simulink model "vehicleModel"  (R2022a)
settings: Solver=ode4  StartTime=0.0  StopTime=100  FixedStep=0.01  RelTol=1e-3
model workspace (MAT data in the model file):
  K = 1
  N = [1 1]
  X = 1
(part 1 of 2)
settings Model: Creator=82106  LastModifiedBy=user
settings ModelReferenceCC: EnableRefExpFcnMdlSchedulingChecks=off
settings RTWCC: Description=Generic Real-Time Target

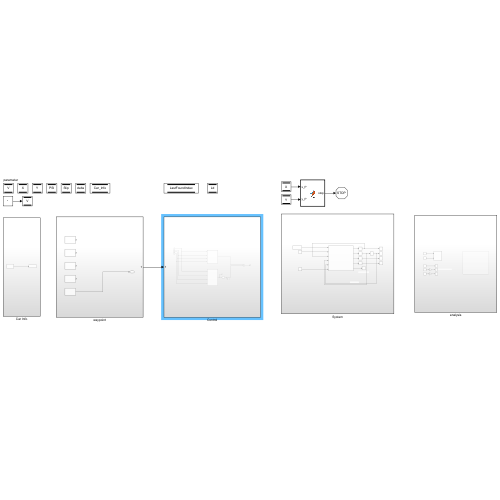
[thumbnail: Simulink's stored preview of the top-level diagram]
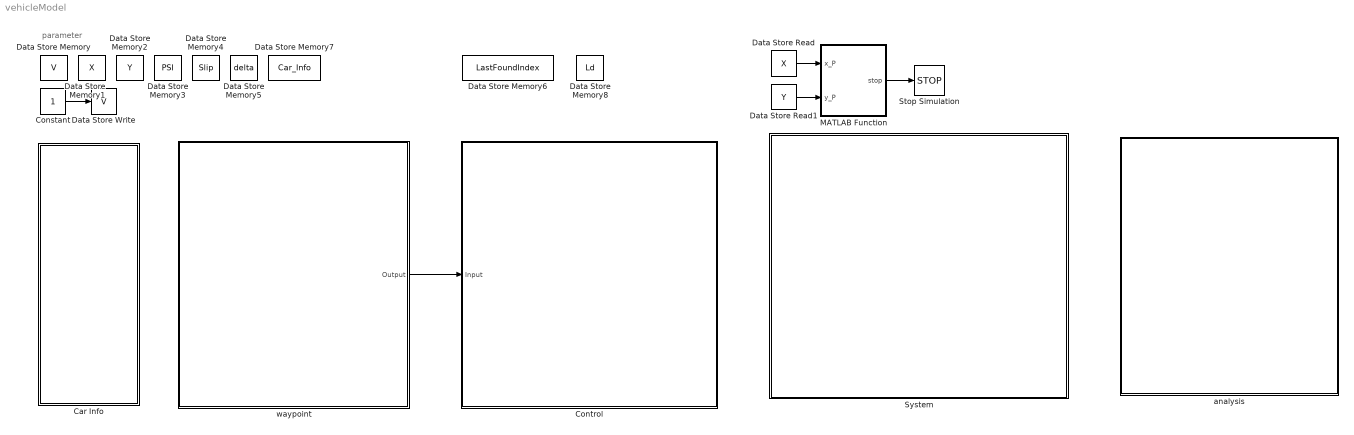
== system vehicleModel ==
  note: parameter
  Car Info : Subsystem
  Constant : Constant
  Control : Subsystem
  Data Store Memory : DataStoreMemory  DataStoreName=V  WriteAfterWriteMsg=warning  ShowAdditionalParam=off
  Data Store Memory1 : DataStoreMemory  DataStoreName=X  WriteAfterWriteMsg=warning  ShowAdditionalParam=off
  Data Store Memory2 : DataStoreMemory  DataStoreName=Y  WriteAfterWriteMsg=warning  ShowAdditionalParam=off
  Data Store Memory3 : DataStoreMemory  DataStoreName=PSI  WriteAfterWriteMsg=warning  ShowAdditionalParam=off
  Data Store Memory4 : DataStoreMemory  DataStoreName=Slip  WriteAfterWriteMsg=warning  ShowAdditionalParam=off
  Data Store Memory5 : DataStoreMemory  DataStoreName=delta  WriteAfterWriteMsg=warning  ShowAdditionalParam=off
  Data Store Memory6 : DataStoreMemory  DataStoreName=LastFoundIndex  WriteAfterWriteMsg=warning  InitialValue=1  ShowAdditionalParam=off
  Data Store Memory7 : DataStoreMemory  DataStoreName=Car_Info  WriteAfterWriteMsg=warning  ShowAdditionalParam=off  Dimensions=6
  Data Store Memory8 : DataStoreMemory  DataStoreName=Ld  WriteAfterWriteMsg=warning  InitialValue=3  ShowAdditionalParam=off
  Data Store Read : DataStoreRead  DataStoreName=X  IndexOptions=Index vector (dialog)  Indices=1  OutputSizes=1
  Data Store Read1 : DataStoreRead  DataStoreName=Y  IndexOptions=Index vector (dialog)  Indices=1  OutputSizes=1
  Data Store Write : DataStoreWrite  DataStoreName=V  IndexOptions=Index vector (dialog)  Indices=1  OutputSizes=1
  MATLAB Function : MATLAB Function  TreatAsAtomicUnit=on
  Stop Simulation : Stop
  System : Subsystem
  analysis : Subsystem
  waypoint : Subsystem
  wires:
  Constant/1 -> Data Store Write/1
  waypoint/1(Output) -> Control/1(Input)
  Data Store Read/1 -> MATLAB Function/1(x_P)
  MATLAB Function/1(stop) -> Stop Simulation/1
  Data Store Read1/1 -> MATLAB Function/2(y_P)

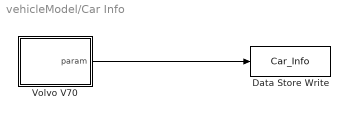
== system vehicleModel/Car Info ==
  Data Store Write : DataStoreWrite  DataStoreName=Car_Info  IndexOptions=Index vector (dialog)  Indices=1  OutputSizes=1
  Volvo V70 : MATLAB Function  TreatAsAtomicUnit=on
  wires:
  Volvo V70/1(param) -> Data Store Write/1

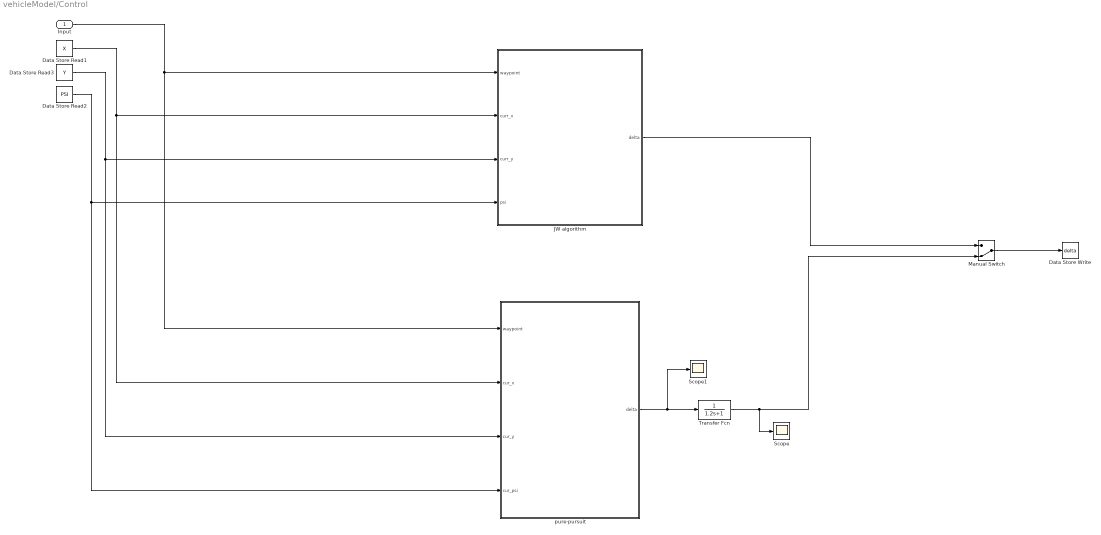
== system vehicleModel/Control ==
  Input : Inport
  Data Store Read1 : DataStoreRead  DataStoreName=X  IndexOptions=Index vector (dialog)  Indices=1  OutputSizes=1
  Data Store Read2 : DataStoreRead  DataStoreName=PSI  IndexOptions=Index vector (dialog)  Indices=1  OutputSizes=1
  Data Store Read3 : DataStoreRead  DataStoreName=Y  IndexOptions=Index vector (dialog)  Indices=1  OutputSizes=1
  Data Store Write : DataStoreWrite  DataStoreName=delta  IndexOptions=Index vector (dialog)  Indices=1  OutputSizes=1
  JW algorithm : Subsystem
  Manual Switch : ManualSwitch  CurrentSetting=0
  Scope : Scope
  Scope1 : Scope
  Transfer Fcn : TransferFcn  Denominator=[1.2 1]
  pure-pursuit : Subsystem
  wires:
  Input/1 -> pure-pursuit/1(waypoint), JW algorithm/1(waypoint)
  Data Store Read2/1 -> pure-pursuit/4(cur_psi), JW algorithm/4(psi)
  Data Store Read3/1 -> pure-pursuit/3(cur_y), JW algorithm/3(curr_y)
  Data Store Read1/1 -> pure-pursuit/2(cur_x), JW algorithm/2(curr_x)
  JW algorithm/1(delta) -> Manual Switch/1
  pure-pursuit/1(delta) -> Scope1/1, Transfer Fcn/1
  Manual Switch/1 -> Data Store Write/1
  Transfer Fcn/1 -> Scope/1, Manual Switch/2

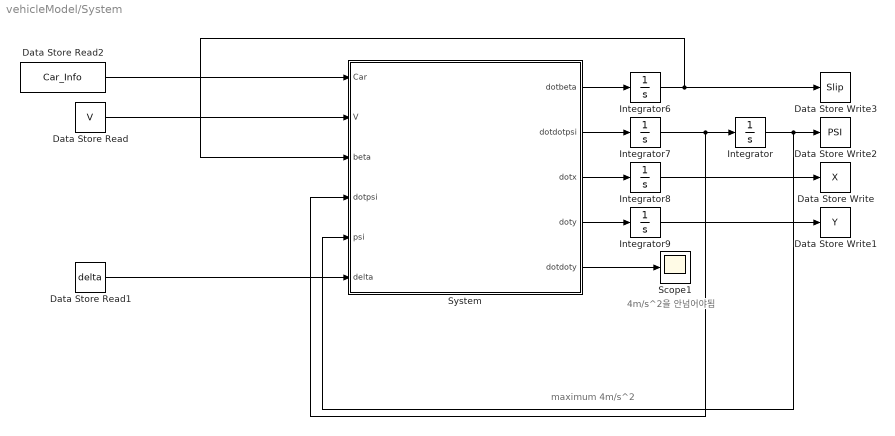
== system vehicleModel/System ==
  note: 4m/s^2을 안넘어야됨
  note: maximum 4m/s^2
  Data Store Read : DataStoreRead  DataStoreName=V  IndexOptions=Index vector (dialog)  Indices=1  OutputSizes=1
  Data Store Read1 : DataStoreRead  DataStoreName=delta  IndexOptions=Index vector (dialog)  Indices=1  OutputSizes=1
  Data Store Read2 : DataStoreRead  DataStoreName=Car_Info  IndexOptions=Index vector (dialog)  Indices=1  OutputSizes=1
  Data Store Write : DataStoreWrite  DataStoreName=X  IndexOptions=Index vector (dialog)  Indices=1  OutputSizes=1
  Data Store Write1 : DataStoreWrite  DataStoreName=Y  IndexOptions=Index vector (dialog)  Indices=1  OutputSizes=1
  Data Store Write2 : DataStoreWrite  DataStoreName=PSI  IndexOptions=Index vector (dialog)  Indices=1  OutputSizes=1
  Data Store Write3 : DataStoreWrite  DataStoreName=Slip  IndexOptions=Index vector (dialog)  Indices=1  OutputSizes=1
  Integrator : Integrator
  Integrator6 : Integrator
  Integrator7 : Integrator
  Integrator8 : Integrator  InitialCondition=1
  Integrator9 : Integrator  InitialCondition=1
  Scope1 : Scope
  System : MATLAB Function  TreatAsAtomicUnit=on
  wires:
  System/5(dotdoty) -> Scope1/1
  System/2(dotdotpsi) -> Integrator7/1
  Integrator9/1 -> Data Store Write1/1
  Integrator6/1 -> System/3(beta), Data Store Write3/1
  Data Store Read/1 -> System/2(V)
  Integrator/1 -> Data Store Write2/1, System/5(psi)
  System/4(doty) -> Integrator9/1
  System/3(dotx) -> Integrator8/1
  Integrator7/1 -> System/4(dotpsi), Integrator/1
  System/1(dotbeta) -> Integrator6/1
  Data Store Read2/1 -> System/1(Car)
  Integrator8/1 -> Data Store Write/1
  Data Store Read1/1 -> System/6(delta)

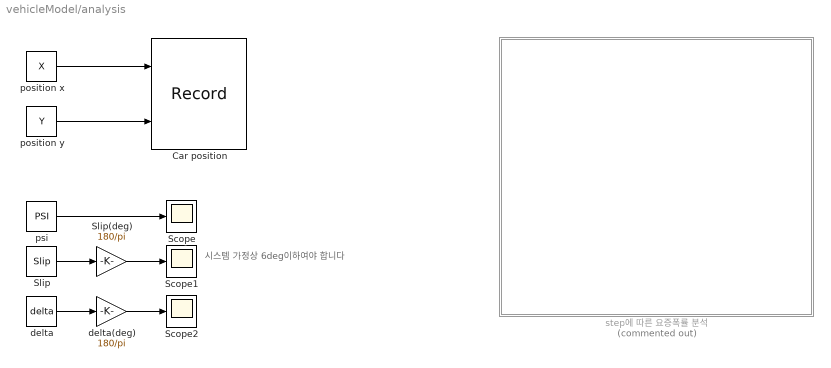
== system vehicleModel/analysis ==
  note: 시스템 가정상 6deg이하여야 합니다
  Car position : Record  FileSettingsInternal="{\"entries\":[{\"content\":{\"excelSettings\":{\"content\":{},\"type\":\"Streamout.ExcelSettings\"}},\"type\":\"Streamout.FileSettingStorage\",\"uuid\":\"dac2e031-e7b2-4fcf-a58f-8ca8c39981c0\"}],\"packageUris\":[\"http://schema.mathworks.com/mf0/streamout_blocks/R2020a\"],\"version\":\"1.0\"}"  Layout=[1 1]  SignalsInternal="{\"entries\":[{\"content\":{\"signals\":[{\"content\":{\"blockPath\":[\"vehicleModel/analysis/Car position\"],\"channel\":[],\"dimensions\":[1],\"domain\":\"vehicleModel/analysis/Car position\",\"lineColor\":\"#a2142f\",\"plots\":[],\"port\":1,\"sid\":[\"\"],\"signalID\":1105,\"signalName\":\"position x\"},\"type\":\"RecordBlkView.Signal\",\"uuid\":\"3ba0c8e4-d376-4e94-8844-daf1410684dd\"},{\"content\":{\"blockPath\":[\"vehicleModel/analysis/Car position\"],\"channel\":[],\"dimensions\":[1],\"domain\":\"vehicleModel/analysis/Car position\",\"lineColor\":\"#139fff\",\"plots\":[1],\"port\":2,\"sid\":[\"\"],\"signalID\":1109,\"signalName\":\"position y\"},\"type\":\"RecordBlkView.Signal\",\"uuid\":\"fbcaf7b4-362f-417e-84a3-3c3b3bc75f13\"}]},\"type\":\"RecordBlkView.InputSignals\",\"uuid\":\"d27d3567-7b96-48c0-b7eb-1a5b4245cb3a\"}],\"packageUris\":[\"http://schema.mathworks.com/mf0/streamout_blocks/R2020a\"],\"version\":\"1.0\"}"  VisualizationBindings="{\"xyplotplugin\":{\"info\":[{\"series\":[{\"bindingParametersList\":[{\"parameter\":\"Y-Axis\",\"signalID\":1109,\"signalName\":\"position y\"}],\"seriesID\":39458}],\"subplotID\":1}]}}"  CompatibilityTag=XY  st=-1
  Scope : Scope
  Scope1 : Scope
  Scope2 : Scope
  Slip : DataStoreRead  DataStoreName=Slip  IndexOptions=Index vector (dialog)  Indices=1  OutputSizes=1
  Slip(deg) : Gain  Gain=180/pi
  delta : DataStoreRead  DataStoreName=delta  IndexOptions=Index vector (dialog)  Indices=1  OutputSizes=1
  delta(deg) : Gain  Gain=180/pi
  position x : DataStoreRead  DataStoreName=X  IndexOptions=Index vector (dialog)  Indices=1  OutputSizes=1
  position y : DataStoreRead  DataStoreName=Y  IndexOptions=Index vector (dialog)  Indices=1  OutputSizes=1
  psi : DataStoreRead  DataStoreName=PSI  IndexOptions=Index vector (dialog)  Indices=1  OutputSizes=1
  step에 따른 요증폭률 분석 : Subsystem  Commented=on
  wires:
  position x/1 -> Car position/1
  position y/1 -> Car position/2
  psi/1 -> Scope/1
  Slip/1 -> Slip(deg)/1
  delta/1 -> delta(deg)/1
  Slip(deg)/1 -> Scope1/1
  delta(deg)/1 -> Scope2/1

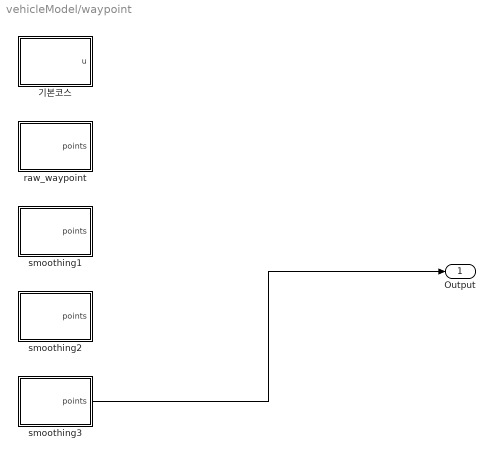
== system vehicleModel/waypoint ==
  raw_waypoint : MATLAB Function  TreatAsAtomicUnit=on
  smoothing1 : MATLAB Function  TreatAsAtomicUnit=on
  smoothing2 : MATLAB Function  TreatAsAtomicUnit=on
  smoothing3 : MATLAB Function  TreatAsAtomicUnit=on
  기본코스 : MATLAB Function  TreatAsAtomicUnit=on
  Output : Outport
  wires:
  smoothing3/1(points) -> Output/1

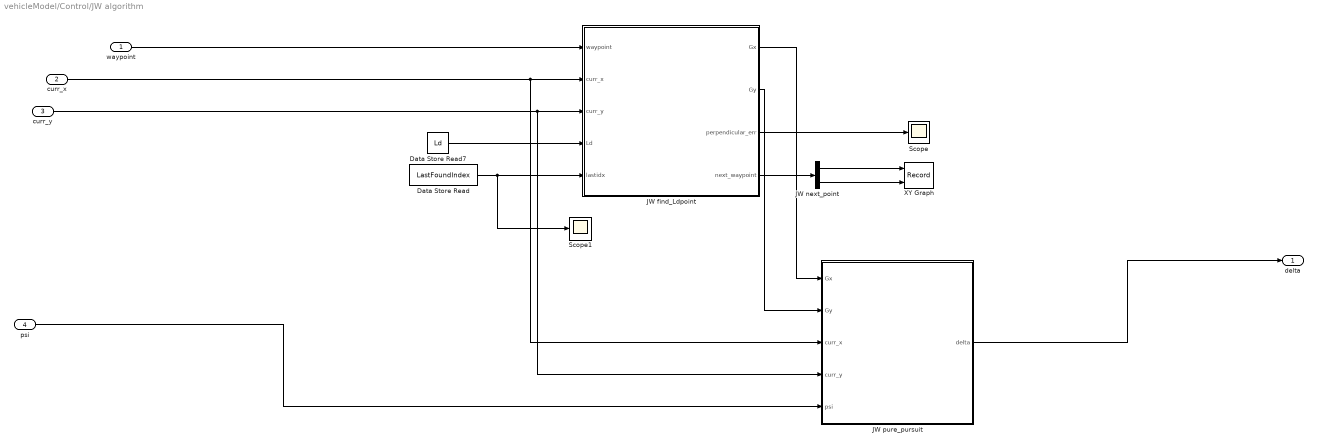
== system vehicleModel/Control/JW algorithm ==
  waypoint : Inport
  curr_x : Inport  Port=2
  curr_y : Inport  Port=3
  psi : Inport  Port=4
  Data Store Read : DataStoreRead  DataStoreName=LastFoundIndex  IndexOptions=Index vector (dialog)  Indices=1  OutputSizes=1
  Data Store Read7 : DataStoreRead  DataStoreName=Ld  IndexOptions=Index vector (dialog)  Indices=1  OutputSizes=1
  JW find_Ldpoint : MATLAB Function  TreatAsAtomicUnit=on
  JW next_point : Demux  Outputs=2
  JW pure_pursuit : MATLAB Function  TreatAsAtomicUnit=on
  Scope : Scope
  Scope1 : Scope
  XY Graph : Record  FileSettingsInternal="{\"entries\":[{\"content\":{\"excelSettings\":{\"content\":{},\"type\":\"Streamout.ExcelSettings\"}},\"type\":\"Streamout.FileSettingStorage\",\"uuid\":\"5d487491-5826-44ea-8ea9-31df16873960\"}],\"packageUris\":[\"http://schema.mathworks.com/mf0/streamout_blocks/R2020a\"],\"version\":\"1.0\"}"  Layout=[1 1]  SignalsInternal="{\"entries\":[{\"content\":{\"signals\":[{\"content\":{\"blockPath\":[\"vehicleModel/Control/JW algorithm/XY Graph\"],\"channel\":[],\"dimensions\":[1,1],\"domain\":\"vehicleModel/Control/JW algorithm/XY Graph\",\"lineColor\":\"#a2142f\",\"plots\":[1],\"port\":1,\"sid\":[\"\"],\"signalID\":1081,\"signalName\":\"JW next_point:1\"},\"type\":\"RecordBlkView.Signal\",\"uuid\":\"1ddf7889-0221-4b01-90d1-93be453a52dd\"},{\"content\":{\"blockPath\":[\"vehicleModel/Control/JW algorithm/XY Graph\"],\"channel\":[],\"dimensions\":[1,1],\"domain\":\"vehicleModel/Control/JW algorithm/XY Graph\",\"lineColor\":\"#b746ff\",\"plots\":[1],\"port\":2,\"sid\":[\"\"],\"signalID\":1085,\"signalName\":\"JW next_point:2\"},\"type\":\"RecordBlkView.Signal\",\"uuid\":\"e3f35186-845d-4813-bc98-4cde5809bf14\"}]},\"type\":\"RecordBlkView.InputSignals\",\"uuid\":\"1f1c30ac-f342-45da-9a67-17280c85dbc6\"}],\"packageUris\":[\"http://schema.mathworks.com/mf0/streamout_blocks/R2020a\"],\"version\":\"1.0\"}"  VisualizationBindings="{\"xyplotplugin\":{\"info\":[{\"series\":[{\"bindingParametersList\":[{\"parameter\":\"X-Axis\",\"signalID\":1081,\"signalName\":\"JW next_point:1\"},{\"parameter\":\"Y-Axis\",\"signalID\":1085,\"signalName\":\"JW next_point:2\"}],\"seriesID\":58780}],\"subplotID\":1}]}}"  CompatibilityTag=XY
  delta : Outport
  wires:
  JW find_Ldpoint/1(Gx) -> JW pure_pursuit/1(Gx)
  curr_x/1 -> JW pure_pursuit/3(curr_x), JW find_Ldpoint/2(curr_x)
  curr_y/1 -> JW pure_pursuit/4(curr_y), JW find_Ldpoint/3(curr_y)
  psi/1 -> JW pure_pursuit/5(psi)
  Data Store Read7/1 -> JW find_Ldpoint/4(Ld)
  JW find_Ldpoint/2(Gy) -> JW pure_pursuit/2(Gy)
  JW pure_pursuit/1(delta) -> delta/1
  Data Store Read/1 -> Scope1/1, JW find_Ldpoint/5(lastidx)
  waypoint/1 -> JW find_Ldpoint/1(waypoint)
  JW find_Ldpoint/3(perpendicular_err) -> Scope/1
  JW find_Ldpoint/4(next_waypoint) -> JW next_point/1
  JW next_point/1 -> XY Graph/1
  JW next_point/2 -> XY Graph/2

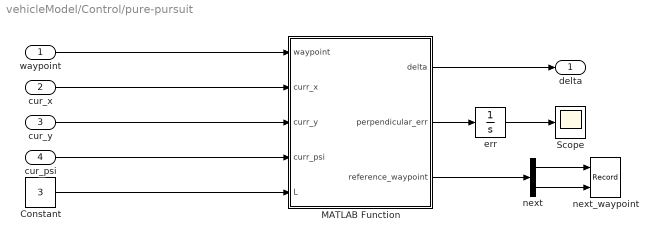
== system vehicleModel/Control/pure-pursuit ==
  waypoint : Inport
  cur_x : Inport  Port=2
  cur_y : Inport  Port=3
  cur_psi : Inport  Port=4
  Constant : Constant  Value=3
  MATLAB Function : MATLAB Function  TreatAsAtomicUnit=on
  Scope : Scope
  err : Integrator
  next : Demux  Outputs=2
  next_waypoint : Record  FileSettingsInternal="{\"entries\":[{\"content\":{\"excelSettings\":{\"content\":{},\"type\":\"Streamout.ExcelSettings\"}},\"type\":\"Streamout.FileSettingStorage\",\"uuid\":\"adb66ec1-1e30-4265-a0c6-ea38e0eb93c2\"}],\"packageUris\":[\"http://schema.mathworks.com/mf0/streamout_blocks/R2020a\"],\"version\":\"1.0\"}"  Layout=[1 1]  SignalsInternal="{\"entries\":[{\"content\":{\"signals\":[{\"content\":{\"blockPath\":[\"vehicleModel/Control/pure-pursuit/next_waypoint\"],\"channel\":[],\"dimensions\":[1,1],\"domain\":\"vehicleModel/Control/pure-pursuit/next_waypoint\",\"lineColor\":\"#64d413\",\"plots\":[],\"port\":1,\"sid\":[\"\"],\"signalID\":1093,\"signalName\":\"next:1\"},\"type\":\"RecordBlkView.Signal\",\"uuid\":\"3e3dcb21-1c56-4110-abf6-f912262a89b0\"},{\"content\":{\"blockPath\":[\"vehicleModel/Control/pure-pursuit/next_waypoint\"],\"channel\":[],\"dimensions\":[1,1],\"domain\":\"vehicleModel/Control/pure-pursuit/next_waypoint\",\"lineColor\":\"#ff13a6\",\"plots\":[],\"port\":2,\"sid\":[\"\"],\"signalID\":1097,\"signalName\":\"next:2\"},\"type\":\"RecordBlkView.Signal\",\"uuid\":\"80a30ef9-14f0-4451-a693-bb1ac6e5dbf5\"}]},\"type\":\"RecordBlkView.InputSignals\",\"uuid\":\"4417b238-cf1e-4cf8-84e5-59b0acfcdd57\"}],\"packageUris\":[\"http://schema.mathworks.com/mf0/streamout_blocks/R2020a\"],\"version\":\"1.0\"}"  VisualizationBindings="{\"xyplotplugin\":{\"info\":[{\"series\":[],\"subplotID\":1}]}}"  CompatibilityTag=XY  st=-1
  delta : Outport
  wires:
  MATLAB Function/1(delta) -> delta/1
  waypoint/1 -> MATLAB Function/1(waypoint)
  Constant/1 -> MATLAB Function/5(L)
  cur_x/1 -> MATLAB Function/2(curr_x)
  cur_y/1 -> MATLAB Function/3(curr_y)
  cur_psi/1 -> MATLAB Function/4(curr_psi)
  MATLAB Function/2(perpendicular_err) -> err/1
  MATLAB Function/3(reference_waypoint) -> next/1
  next/1 -> next_waypoint/1
  next/2 -> next_waypoint/2
  err/1 -> Scope/1

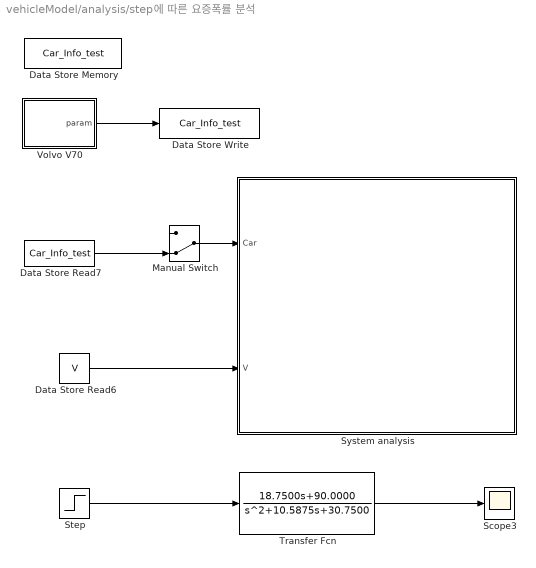
== system vehicleModel/analysis/step에 따른 요증폭률 분석 ==
  Data Store Memory : DataStoreMemory  DataStoreName=Car_Info_test  WriteAfterWriteMsg=warning  ShowAdditionalParam=off  Dimensions=6
  Data Store Read6 : DataStoreRead  DataStoreName=V  IndexOptions=Index vector (dialog)  Indices=1  OutputSizes=1
  Data Store Read7 : DataStoreRead  DataStoreName=Car_Info_test  IndexOptions=Index vector (dialog)  Indices=1  OutputSizes=1
  Data Store Write : DataStoreWrite  DataStoreName=Car_Info_test  IndexOptions=Index vector (dialog)  Indices=1  OutputSizes=1
  Manual Switch : ManualSwitch  CurrentSetting=0
  Scope3 : Scope
  Step : Step  SampleTime=0
  System analysis : MATLAB Function  TreatAsAtomicUnit=on
  Transfer Fcn : TransferFcn  Numerator="[18.7500   90.0000]"  Denominator="[1.0000   10.5875   30.7500]"
  Volvo V70 : MATLAB Function  TreatAsAtomicUnit=on
  wires:
  Step/1 -> Transfer Fcn/1
  Data Store Read7/1 -> Manual Switch/2
  Transfer Fcn/1 -> Scope3/1
  Data Store Read6/1 -> System analysis/2(V)
  Manual Switch/1 -> System analysis/1(Car)
  Volvo V70/1(param) -> Data Store Write/1

== matlab function vehicleModel/waypoint/smoothing2 ==
  data: points output
function points = waypoint()

points = [
    1	1
1.11704648353462	1.09353971332660
1.23753282262680	1.18288758455006
1.35801916171897	1.27223545577353
1.47850550081115	1.36158332699700
1.59899183990332	1.45093119822047
1.71947817899550	1.54027906944393
1.83824947077548	1.63177819792942
1.93195904490435	1.74818382989704
1.97773993586061	2.14778137751352
1.93589683576808	2.29182704726671
1.89405373567555	2.43587271701991
1.85782290823178	2.58124470101719
1.86069549057951	2.73065522175738
1.90759360128083	2.87254363795068
2.10606601717798	3.10606601717798
2.21213203435596	3.21213203435596
2.31819805153395	3.31819805153395
2.42426406871193	3.42426406871193
2.53033008588991	3.53033008588991
2.63639610306789	3.63639610306789
2.74246212024588	3.74246212024587
2.84852813742386	3.84852813742386
3.10606601717798	4.10606601717798
3.21213203435596	4.21213203435596
3.31819805153395	4.31819805153395
3.42426406871193	4.42426406871193
3.53033008588991	4.53033008588991
3.63639610306789	4.63639610306789
3.74246212024588	4.74246212024588
3.84852813742386	4.84852813742386
4.11704648353462	5.09353971332660
4.23753282262680	5.18288758455006
4.35801916171897	5.27223545577353
4.47850550081115	5.36158332699700
4.59899183990332	5.45093119822047
4.71947817899550	5.54027906944393
4.83824947077548	5.63177819792942
4.93195904490435	5.74818382989704
5	6.15000000000000
5	6.30000000000000
5	6.45000000000000
5	6.60000000000000
5	6.75000000000000
5	7.15000000000000
5	7.30000000000000
5	7.45000000000000
5	7.60000000000000
5	7.75000000000000
4.97773993586061	8.14778137751352
4.93589683576808	8.29182704726671
4.89405373567555	8.43587271701991
4.85782290823178	8.58124470101719
4.86069549057951	8.73065522175738
4.90759360128083	8.87254363795068
5.10606601717798	9.10606601717798
5.21213203435596	9.21213203435596
5.31819805153395	9.31819805153395
5.42426406871193	9.42426406871193
5.53033008588991	9.53033008588991
5.63639610306789	9.63639610306789
5.74246212024588	9.74246212024588
5.84852813742386	9.84852813742386
6.10606601717798	10.1060660171780
6.21213203435596	10.2121320343560
6.31819805153395	10.3181980515339
6.42426406871193	10.4242640687119
6.53033008588991	10.5303300858899
6.63639610306789	10.6363961030679
6.74246212024588	10.7424621202459
6.84852813742386	10.8485281374239
7.09353971332660	11.1170464835346
7.18288758455007	11.2375328226268
7.27223545577353	11.3580191617190
7.36158332699700	11.4785055008112
7.45093119822047	11.5989918399033
7.54027906944393	11.7194781789955
7.63177819792942	11.8382494707755
7.74818382989704	11.9319590449044
8.14778137751352	11.9777399358606
8.29182704726671	11.9358968357681
8.43587271701991	11.8940537356756
8.58124470101719	11.8578229082318
8.73065522175738	11.8606954905795
8.87254363795068	11.9075936012808
9.10606601717798	12.1060660171780
9.21213203435596	12.2121320343560
9.31819805153395	12.3181980515339
9.42426406871193	12.4242640687119
9.53033008588991	12.5303300858899
9.63639610306789	12.6363961030679
9.74246212024588	12.7424621202459
9.84852813742386	12.8485281374239
10.1060660171780	13.1060660171780
10.2121320343560	13.2121320343560
10.3181980515339	13.3181980515339
10.4242640687119	13.4242640687119
10.5303300858899	13.5303300858899
10.6363961030679	13.6363961030679
10.7424621202459	13.7424621202459
10.8485281374239	13.8485281374239
11.0935397133266	14.1170464835346
11.1828875845501	14.2375328226268
11.2722354557735	14.3580191617190
11.3615833269970	14.4785055008112
11.4509311982205	14.5989918399033
11.5402790694439	14.7194781789955
11.6317781979294	14.8382494707755
11.7481838298970	14.9319590449044
12.1500000000000	15
12.3000000000000	15
12.4500000000000	15
12.6000000000000	15
12.7500000000000	15
13.1500000000000	15
13.3000000000000	15
13.4500000000000	15
13.6000000000000	15
13.7500000000000	15
14.1500000000000	15
14.3000000000000	15
14.4500000000000	15
14.6000000000000	15
14.7500000000000	15
15.1477813775135	14.9777399358606
15.2918270472667	14.9358968357681
15.4358727170199	14.8940537356756
15.5812447010172	14.8578229082318
15.7306552217574	14.8606954905795
15.8725436379507	14.9075936012808
16.1060660171780	15.1060660171780
16.2121320343560	15.2121320343560
16.3181980515339	15.3181980515339
16.4242640687119	15.4242640687119
16.5303300858899	15.5303300858899
16.6363961030679	15.6363961030679
16.7424621202459	15.7424621202459
16.8485281374239	15.8485281374239
17.1170464835346	16.0935397133266
17.2375328226268	16.1828875845501
17.3580191617190	16.2722354557735
17.4785055008112	16.3615833269970
17.5989918399033	16.4509311982205
17.7194781789955	16.5402790694439
17.8382494707755	16.6317781979294
17.9319590449044	16.7481838298970
18	17.1500000000000
18	17.3000000000000
18	17.4500000000000
18	17.6000000000000
18	17.7500000000000
17.9777399358606	18.1477813775135
17.9358968357681	18.2918270472667
17.8940537356756	18.4358727170199
17.8578229082318	18.5812447010172
17.8606954905795	18.7306552217574
17.9075936012808	18.8725436379507
18.1060660171780	19.1060660171780
18.2121320343560	19.2121320343560
18.3181980515339	19.3181980515339
18.4242640687119	19.4242640687119
18.5303300858899	19.5303300858899
18.6363961030679	19.6363961030679
18.7424621202459	19.7424621202459
18.8485281374239	19.8485281374239
19.1060660171780	20.1060660171780
19.2121320343560	20.2121320343560
19.3181980515339	20.3181980515339
19.4242640687119	20.4242640687119
19.5303300858899	20.5303300858899
19.6363961030679	20.6363961030679
19.7424621202459	20.7424621202459
19.8485281374239	20.8485281374239
20.1060660171780	21.1060660171780
20.2121320343560	21.2121320343560
20.3181980515339	21.3181980515339
20.4242640687119	21.4242640687119
20.5303300858899	21.5303300858899
20.6363961030679	21.6363961030679
20.7424621202459	21.7424621202459
20.8485281374239	21.8485281374239
21.1060660171780	22.1060660171780
21.2121320343560	22.2121320343560
21.3181980515339	22.3181980515339
21.4242640687119	22.4242640687119
21.5303300858899	22.5303300858899
21.6363961030679	22.6363961030679
21.7424621202459	22.7424621202459
21.8485281374239	22.8485281374239
22.1060660171780	23.1060660171780
22.2121320343560	23.2121320343560
22.3181980515339	23.3181980515339
22.4242640687119	23.4242640687119
22.5303300858899	23.5303300858899
22.6363961030679	23.6363961030679
22.7424621202459	23.7424621202459
22.8485281374239	23.8485281374239
23.1060660171780	24.1060660171780
23.2121320343560	24.2121320343560
23.3181980515339	24.3181980515339
23.4242640687119	24.4242640687119
23.5303300858899	24.5303300858899
23.6363961030679	24.6363961030679
23.7424621202459	24.7424621202459
23.8485281374239	24.8485281374239
24.1060660171780	25.1060660171780
24.2121320343560	25.2121320343560
24.3181980515339	25.3181980515339
24.4242640687119	25.4242640687119
24.5303300858899	25.5303300858899
24.6363961030679	25.6363961030679
24.7424621202459	25.7424621202459
24.8485281374239	25.8485281374239
25.1170464835346	26.0935397133266
25.2375328226268	26.1828875845501
25.3580191617190	26.2722354557735
25.4785055008112	26.3615833269970
25.5989918399033	26.4509311982205
25.7194781789955	26.5402790694439
25.8382494707755	26.6317781979294
25.9319590449044	26.7481838298970
26	27.1500000000000
26	27.3000000000000
26	27.4500000000000
26	27.6000000000000
26	27.7500000000000
26	28.1500000000000
26	28.3000000000000
26	28.4500000000000
26	28.6000000000000
26	28.7500000000000
26	29.1500000000000
26	29.3000000000000
26	29.4500000000000
26	29.6000000000000
26	29.7500000000000
26	30.1500000000000
26	30.3000000000000
26	30.4500000000000
26	30.6000000000000
26	30.7500000000000
26	31.1500000000000
26	31.3000000000000
26	31.4500000000000
26	31.6000000000000
26	31.7500000000000
26	32.1500000000000
26	32.3000000000000
26	32.4500000000000
26	32.6000000000000
26	32.7500000000000
26	33.1500000000000
26	33.3000000000000
26	33.4500000000000
26	33.6000000000000
26	33.7500000000000
26	34.1500000000000
26	34.3000000000000
26	34.4500000000000
26	34.6000000000000
26	34.7500000000000
26	35.1500000000000
26	35.3000000000000
26	35.4500000000000
26	35.6000000000000
26	35.7500000000000
26	36.1500000000000
26	36.3000000000000
26	36.4500000000000
26	36.6000000000000
26	36.7500000000000
26	37.1500000000000
26	37.3000000000000
26	37.4500000000000
26	37.6000000000000
26	37.7500000000000
25.9777399358606	38.1477813775135
25.9358968357681	38.2918270472667
25.8940537356756	38.4358727170199
25.8578229082318	38.5812447010172
25.8606954905795	38.7306552217574
25.9075936012808	38.8725436379507
26.1060660171780	39.1060660171780
26.2121320343560	39.2121320343560
26.3181980515339	39.3181980515340
26.4242640687119	39.4242640687119
26.5303300858899	39.5303300858899
26.6363961030679	39.6363961030679
26.7424621202459	39.7424621202459
26.8485281374239	39.8485281374239
27.1060660171780	40.1060660171780
27.2121320343560	40.2121320343560
27.3181980515339	40.3181980515340
27.4242640687119	40.4242640687119
27.5303300858899	40.5303300858899
27.6363961030679	40.6363961030679
27.7424621202459	40.7424621202459
27.8485281374239	40.8485281374239
28.1170464835346	41.0935397133266
28.2375328226268	41.1828875845501
28.3580191617190	41.2722354557735
28.4785055008112	41.3615833269970
28.5989918399033	41.4509311982205
28.7194781789955	41.5402790694439
28.8382494707755	41.6317781979294
28.9319590449044	41.7481838298970
29	42.1500000000000
29	42.3000000000000
29	42.4500000000000
29	42.6000000000000
29	42.7500000000000
28.9777399358606	43.1477813775135
28.9358968357681	43.2918270472667
28.8940537356756	43.4358727170199
28.8578229082318	43.5812447010172
28.8606954905795	43.7306552217574
28.9075936012808	43.8725436379507
29.1060660171780	44.1060660171780
29.2121320343560	44.2121320343560
29.3181980515339	44.3181980515340
29.4242640687119	44.4242640687119
29.5303300858899	44.5303300858899
29.6363961030679	44.6363961030679
29.7424621202459	44.7424621202459
29.8485281374239	44.8485281374239
30.1060660171780	45.1060660171780
30.2121320343560	45.2121320343560
30.3181980515339	45.3181980515340
30.4242640687119	45.4242640687119
30.5303300858899	45.5303300858899
30.6363961030679	45.6363961030679
30.7424621202459	45.7424621202459
30.8485281374239	45.8485281374239
31.1060660171780	46.1060660171780
31.2121320343560	46.2121320343560
31.3181980515339	46.3181980515340
31.4242640687119	46.4242640687119
31.5303300858899	46.5303300858899
31.6363961030679	46.6363961030679
31.7424621202459	46.7424621202459
31.8485281374239	46.8485281374239
32.1060660171780	47.1060660171780
32.2121320343560	47.2121320343560
32.3181980515340	47.3181980515340
32.4242640687119	47.4242640687119
32.5303300858899	47.5303300858899
32.6363961030679	47.6363961030679
32.7424621202459	47.7424621202459
32.8485281374239	47.8485281374239
33.0935397133266	48.1170464835346
33.1828875845501	48.2375328226268
33.2722354557735	48.3580191617190
33.3615833269970	48.4785055008111
33.4509311982205	48.5989918399033
33.5402790694439	48.7194781789955
33.6317781979294	48.8382494707755
33.7481838298970	48.9319590449044
34.1500000000000	49
34.3000000000000	49
34.4500000000000	49
34.6000000000000	49
34.7500000000000	49
35.1500000000000	49
35.3000000000000	49
35.4500000000000	49
35.6000000000000	49
35.7500000000000	49
36.1500000000000	49
36.3000000000000	49
36.4500000000000	49
36.6000000000000	49
36.7500000000000	49
37.1500000000000	49
37.3000000000000	49
37.4500000000000	49
37.6000000000000	49
37.7500000000000	49
38.1500000000000	49
38.3000000000000	49
38.4500000000000	49
38.6000000000000	49
38.7500000000000	49
39.1500000000000	49
39.3000000000000	49
39.4500000000000	49
39.6000000000000	49
39.7500000000000	49
40.1500000000000	49
40.3000000000000	49
40.4500000000000	49
40.6000000000000	49
40.7500000000000	49
41.1500000000000	49
41.3000000000000	49
41.4500000000000	49
41.6000000000000	49
41.7500000000000	49
42.1500000000000	49
42.3000000000000	49
42.4500000000000	49
42.6000000000000	49
42.7500000000000	49
43.1500000000000	49
43.3000000000000	49
43.4500000000000	49
43.6000000000000	49
43.7500000000000	49
44.1500000000000	49
44.3000000000000	49
44.4500000000000	49
44.6000000000000	49
44.7500000000000	49
45.1477813775135	48.9777399358606
45.2918270472667	48.9358968357681
45.4358727170199	48.8940537356756
45.5812447010172	48.8578229082318
45.7306552217574	48.8606954905795
45.8725436379507	48.9075936012808
46.1060660171780	49.1060660171780
46.2121320343560	49.2121320343560
46.3181980515340	49.3181980515340
46.4242640687119	49.4242640687119
46.5303300858899	49.5303300858899
46.6363961030679	49.6363961030679
46.7424621202459	49.7424621202459
46.8485281374239	49.8485281374239
47.1060660171780	50.1060660171780
47.2121320343560	50.2121320343560
47.3181980515340	50.3181980515340
47.4242640687119	50.4242640687119
47.5303300858899	50.5303300858899
47.6363961030679	50.6363961030679
47.7424621202459	50.7424621202459
47.8485281374239	50.8485281374239
48.0935397133266	51.1170464835346
48.1828875845501	51.2375328226268
48.2722354557735	51.3580191617190
48.3615833269970	51.4785055008111
48.4509311982205	51.5989918399033
48.5402790694439	51.7194781789955
48.6317781979294	51.8382494707755
48.7481838298970	51.9319590449044
49.1500000000000	52
49.3000000000000	52
49.4500000000000	52
49.6000000000000	52
49.7500000000000	52
50.1500000000000	52
50.3000000000000	52
50.4500000000000	52
50.6000000000000	52
50.7500000000000	52
51.1477813775135	51.9777399358606
51.2918270472667	51.9358968357681
51.4358727170199	51.8940537356756
51.5812447010172	51.8578229082318
51.7306552217574	51.8606954905795
51.8725436379507	51.9075936012808
52.1060660171780	52.1060660171780
52.2121320343560	52.2121320343560
52.3181980515340	52.3181980515340
52.4242640687119	52.4242640687119
52.5303300858899	52.5303300858899
52.6363961030679	52.6363961030679
52.7424621202459	52.7424621202459
52.8485281374239	52.8485281374239
53.1060660171780	53.1060660171780
53.2121320343560	53.2121320343560
53.3181980515340	53.3181980515340
53.4242640687119	53.4242640687119
53.5303300858899	53.5303300858899
53.6363961030679	53.6363961030679
53.7424621202459	53.7424621202459
53.8485281374239	53.8485281374239
54.1060660171780	54.1060660171780
54.2121320343560	54.2121320343560
54.3181980515340	54.3181980515340
54.4242640687119	54.4242640687119
54.5303300858899	54.5303300858899
54.6363961030679	54.6363961030679
54.7424621202459	54.7424621202459
54.8485281374239	54.8485281374239
55.1060660171780	55.1060660171780
55.2121320343560	55.2121320343560
55.3181980515340	55.3181980515340
55.4242640687119	55.4242640687119
55.5303300858899	55.5303300858899
55.6363961030679	55.6363961030679
55.7424621202459	55.7424621202459
55.8485281374239	55.8485281374239
56.1060660171780	56.1060660171780
56.2121320343560	56.2121320343560
56.3181980515340	56.3181980515340
56.4242640687119	56.4242640687119
56.5303300858899	56.5303300858899
56.6363961030679	56.6363961030679
56.7424621202459	56.7424621202459
56.8485281374239	56.8485281374239
57.1052085736752	57.1069165221417
57.2104053055217	57.2138447579301
57.3156020373681	57.3207729937185
57.4207987692146	57.4277012295069
57.5259955010611	57.5346294652953
57.6311922329076	57.6415577010837
57.7363889647541	57.7484859368721
57.8415856966006	57.8554141726605
58	58];

end
